simulink model "demo_ifft"  (R2023a)
settings: Solver=FixedStepDiscrete  StartTime=0.0  StopTime=dspb_ifft.SimulationTime  FixedStep=1  RelTol=1e-3  EnableMultiTasking=on
PreLoadFcn:
  | warning off Simulink:Commands:SetParamLinkChangeWarn
  | warning off Simulink:Commands:LoadMdlParameterizedLink
  | warning off Simulink:SL_SetParamLinkChangeWarn
  | warning off Simulink:SL_LoadMdlParameterizedLink
  | setup_demo_ifft;
InitFcn:
  | setup_demo_ifft;
StopFcn:
  | analyze_subchannel_fft(...
  |      dspb_ifft.FFTsize, ...
  |      dspb_ifft.subchannels, ...
  |      dspb_ifft.IFFT, ...
  |      dspb_ifft.bit_reversed, ...
  |      dspb_ifft.bit_reversed, ...
  |      v_in, chan_in,  x_in, ...
  |      v_out,chan_out, z_out);
undefined symbols (not defined in the file or in its folder): dspb_ifft, value
libraries: DSPBAPrim x8, DSPBABase x4, DSPBAVectorUtil x3, simulink x3, DspbAdvFftLibrary x2
Description:
  | This design example implements an Inverse Fast Fourier Transform.
settings Model: Creator=lrigby  LastModifiedBy=5g
settings SolverCC: AlgebraicLoopSolver=TrustRegion
settings DataIOCC: LimitDataPoints=on  SaveFormat=Array  SignalLoggingSaveFormat=ModelDataLogs  ReturnWorkspaceOutputs=off
settings OptimizationCC: ExpressionDepthLimit=2147483647  InitFltsAndDblsToZero=on  LifeSpan=inf
settings DebuggingCC: SaveWithParameterizedLinksMsg=none  UnderspecifiedInitializationDetection=Classic  MergeDetectMultiDrivingBlocksExec=none  SignalResolutionControl=TryResolveAllWithWarning  SolverPrmCheckMsg=warning  ParameterPrecisionLossMsg=none  FcnCallInpInsideContextMsg=warning  UnconnectedInputMsg=warning  UnconnectedOutputMsg=warning  UnconnectedLineMsg=warning  StateNameClashWarn=warning  SFUnexpectedBacktrackingDiag=warning  SFNoUnconditionalDefaultTransitionDiag=warning  SFExecutionAtInitializationDiag=none  ArithmeticOperatorsInVariantConditions=warning
settings HardwareCC: ProdBitPerPointer=32  ProdBitPerSizeT=32  ProdBitPerPtrDiffT=32  ProdLargestAtomicFloat=None  ProdIntDivRoundTo=Undefined  ProdEndianess=Unspecified  ProdWordSize=32  ProdHWDeviceType=ASIC/FPGA  TargetBitPerLong=64  TargetBitPerPointer=64  TargetBitPerSizeT=64  TargetBitPerPtrDiffT=64  TargetLongLongMode=on  TargetIntDivRoundTo=Zero  TargetEndianess=LittleEndian  TargetWordSize=64  TargetHWDeviceType=MATLAB Host  ProdEqTarget=off
settings ModelReferenceCC: PropagateSignalLabelsOutOfModel=off
settings SFSimCC: SimUseLocalCustomCode=off  SimParseCustomCode=off  CustomCodeUndefinedFunction=UseInterfaceOnly
settings RTWCC: RTWUseLocalCustomCode=off
settings CodeAppCC: StateflowObjectComments=on
settings GRTTargetCC: TargetFcnLib=ansi_tfl_tmw.mat  TargetLangStandard=C89/C90 (ANSI)  CombineOutputUpdateFcns=off  GRTInterface=on
settings ConfigComp: CovMetricSettings=dw  CovSaveCumulativeToWorkspaceVar=on  CovSaveSingleToWorkspaceVar=on  CovExternalEMLEnable=off

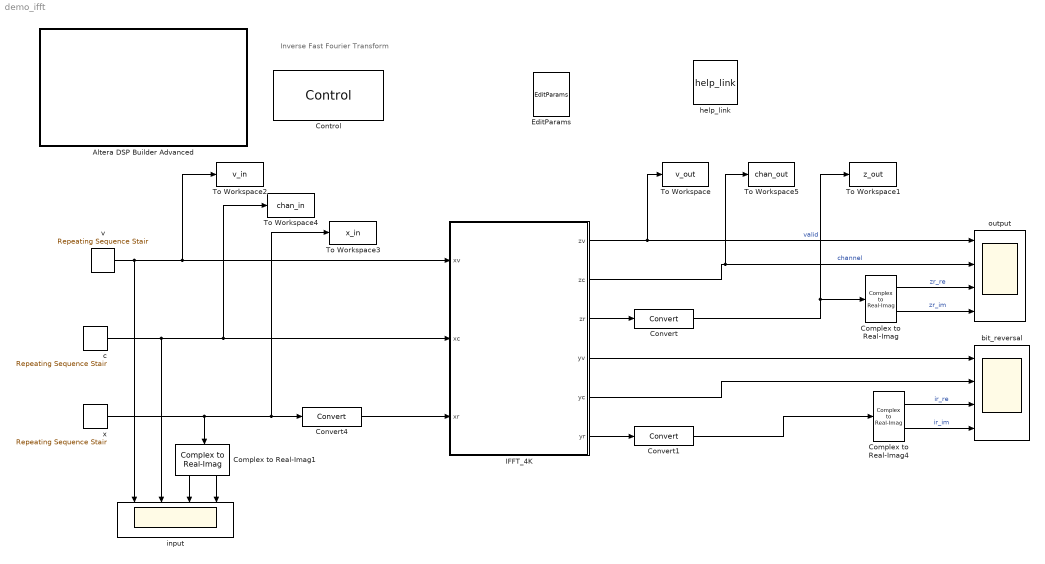
== system demo_ifft ==
  note: Inverse Fast Fourier Transform
  Altera DSP Builder Advanced : Subsystem  mask(DSP Builder Advanced Blockset Ignored Block){}
      settings: OpenFcn=web('http://www.altera.com', '-new');
      mask Display: image(imread('intellogo.tif'));
  Complex to Real-Imag : DSPBAVectorUtil/Complex to Real-Imag
  Complex to Real-Imag1 : DSPBAVectorUtil/Complex to Real-Imag
  Complex to Real-Imag4 : DSPBAVectorUtil/Complex to Real-Imag
  Control : DSPBABase/Control  generate=on  language=VHDL  destination=../rtl  make_full_path=off  path_is_relative=on  autotestbench=on  signaldepth=2  coveragetestbench=off  logs=off  spacewidth=2  spacenum=1  addrwidth=10  datawidth=16  dataendian=Big Endian  hierarchicalnames=on  ramThresholdBits=-1  distRamThresholdBits=-1  mlabThresholdBits=-1  hardMultiplierThresholdLuts=-1  version=20090407  errorOnChanMismatch=1  errorOnGPIOMismatch=0  importModelsimResults=0  cycleAccurate=off  reinterpretCastMult=off  paramFile=demo_ifft_params.xml
  Convert : DSPBAPrim/Convert  primtype=convert  nInputs=1  nOutputs=1  omode=double  otype=sfix(16)  scale=2^-15  rndmethod=Unbiased  factor=1  satmethod=None  shift_vec=[0 1 2 -1]  value=round([0:255]/17)  inPortNames=[' '; ' ';]  outPortNames=[' '; 'c']  dspbaimage=dspba_prim_wide.svg  text=fprintf('convert');  style=Optimised  visibilities=8+64+256+2^17  clipdetect=off  floatPrecision=float32_m23  advOptions=[]  version=20211007
  Convert1 : DSPBAPrim/Convert  primtype=convert  nInputs=1  nOutputs=1  omode=double  otype=sfix(16)  scale=2^-15  rndmethod=Unbiased  factor=1  satmethod=None  shift_vec=[0 1 2 -1]  value=round([0:255]/17)  inPortNames=[' '; ' ';]  outPortNames=[' '; 'c']  dspbaimage=dspba_prim_wide.svg  text=fprintf('convert');  style=Optimised  visibilities=8+64+256+2^17  clipdetect=off  floatPrecision=float32_m23  advOptions=[]  version=20211007
  Convert4 : DSPBAPrim/Convert  primtype=convert  nInputs=1  nOutputs=1  omode=Specify via dialog  otype=sfix(16)  scale=2^-14  rndmethod=Unbiased  factor=1  satmethod=None  shift_vec=[0 1 2 -1]  value=round([0:255]/17)  inPortNames=[' '; ' ';]  outPortNames=[' '; 'c']  dspbaimage=dspba_prim_wide.svg  text=fprintf('convert');  style=Optimised  visibilities=8+64+256+2^17  clipdetect=off  floatPrecision=float32_m23  advOptions=[]  version=20211007
  EditParams : DSPBABase/EditParams  version=20090407
  IFFT_4K : Subsystem
  To Workspace : ToWorkspace  VariableName=v_out  SampleTime=-1
  To Workspace1 : ToWorkspace  VariableName=z_out  SampleTime=-1
  To Workspace2 : ToWorkspace  VariableName=v_in  SampleTime=-1
  To Workspace3 : ToWorkspace  VariableName=x_in  SampleTime=-1
  To Workspace4 : ToWorkspace  VariableName=chan_in  SampleTime=-1
  To Workspace5 : ToWorkspace  VariableName=chan_out  SampleTime=-1
  bit_reversal : Scope  NumInputPorts=4
  c : simulink/Sources/Repeating Sequence Stair  OutValues=dspb_ifft.channel_in  tsamp=dspb_ifft.SampleTime  OutMin=[]  OutMax=[]  OutDataTypeStr=fixdt(0,8,0)  OutputDataTypeScalingMode=Specify via dialog  OutDataType=uint(8)  ConRadixGroup=Use specified scaling  OutScaling=2^-15
  help_link : DSPBABase/help_link  version=20090407
  input : Scope  NumInputPorts=4
  output : Scope  NumInputPorts=4
  v : simulink/Sources/Repeating Sequence Stair  OutValues=dspb_ifft.valid_in  tsamp=dspb_ifft.SampleTime  OutMin=[]  OutMax=[]  OutDataTypeStr=fixdt('boolean')  OutputDataTypeScalingMode=Specify via dialog  OutDataType=fixdt('boolean')  ConRadixGroup=Best Precision: Vector-wise  OutScaling=[]
  x : simulink/Sources/Repeating Sequence Stair  OutValues=dspb_ifft.x_in  tsamp=dspb_ifft.SampleTime  OutMin=[]  OutMax=[]  OutDataTypeStr=double  OutputDataTypeScalingMode=double  OutDataType=dspb_ifft.InputType  ConRadixGroup=Best Precision: Vector-wise  OutScaling=[]
  wires:
  v/1 -> input/1, To Workspace2/1, IFFT_4K/1(xv)
  c/1 -> To Workspace4/1, IFFT_4K/2(xc), input/2
  x/1 -> Complex to Real-Imag1/1, To Workspace3/1, Convert4/1
  IFFT_4K/3(zr) -> Convert/1
  Complex to Real-Imag/1 -> output/3  "zr_re"
  Complex to Real-Imag/2 -> output/4  "zr_im"
  Complex to Real-Imag1/1 -> input/3
  Complex to Real-Imag1/2 -> input/4
  Convert/1 -> Complex to Real-Imag/1, To Workspace1/1
  IFFT_4K/6(yr) -> Convert1/1
  IFFT_4K/1(zv) -> output/1, To Workspace/1  "valid"
  IFFT_4K/2(zc) -> output/2, To Workspace5/1  "channel"
  Convert4/1 -> IFFT_4K/3(xr)
  Convert1/1 -> Complex to Real-Imag4/1
  IFFT_4K/4(yv) -> bit_reversal/1
  IFFT_4K/5(yc) -> bit_reversal/2
  Complex to Real-Imag4/1 -> bit_reversal/3  "ir_re"
  Complex to Real-Imag4/2 -> bit_reversal/4  "ir_im"

== system demo_ifft/Altera DSP Builder Advanced ==

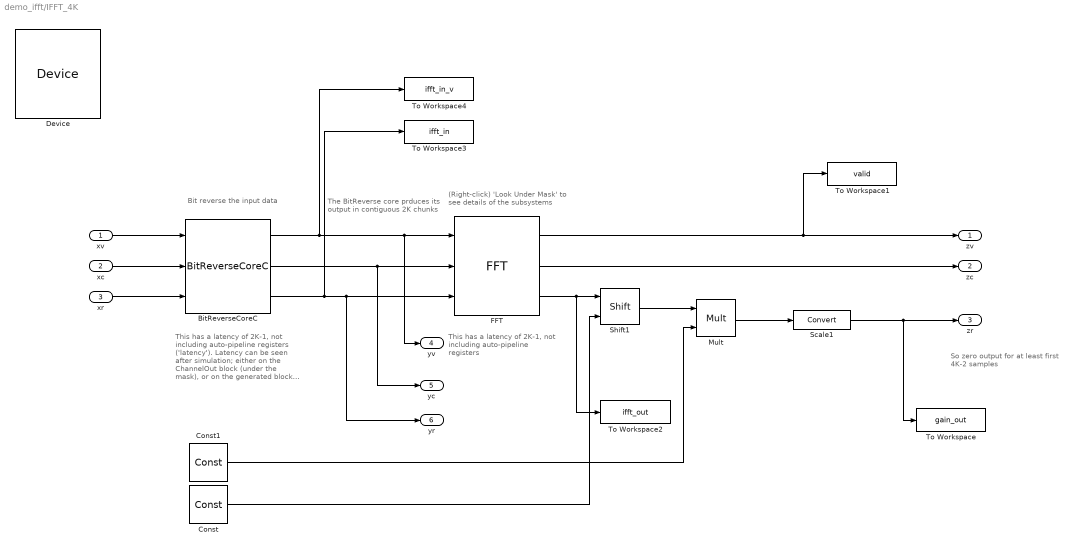
== system demo_ifft/IFFT_4K ==
  note: Bit reverse the input data
  note: This has a latency of 2K-1,
      | not including auto-pipeline
      | registers ('latency'). Latency
      | can be seen after simulation;
      | either on the ChannelOut block
      | (under the mask), or on the
      | generated block help.
  note: This has a latency of 2K-1,
      | not including auto-pipeline
      | registers
  note: So zero output for at
      | least first 4K-2 samples
  note: (Right-click) 'Look Under Mask'
      | to see details of the subsystems
  note: The BitReverse core prduces its
      | output in contiguous 2K chunks
  xv : Inport
  xc : Inport  Port=2
  xr : Inport  Port=3
  BitReverseCoreC : DspbAdvFftLibrary/Radix2/BitReverseCoreC  N=dspb_ifft.FFTsize  subchannels=dspb_ifft.subchannels
      link override ChannelOut: value=1  latency=6  nInputs=dspba_internal_get_channel_ports(gcb, 'inputs')  nOutputs=dspba_internal_get_channel_ports(gcb, 'outputs')  packetBeginEnabled=off  version=20140818
  Const : DSPBAPrim/Const  primtype=const  nInputs=0  nOutputs=1  omode=Specify via dialog  otype=ufix(4)  scale=0  rndmethod=Unbiased  factor=1  satmethod=Symmetric  shift_vec=[0 1 2 -1]  value=12  inPortNames=['+'; '+';]  outPortNames=[' ']  dspbaimage=dspba_prim.svg  text=fprintf('%s', num2str(value));  style=Optimised  visibilities=8 + 1024  floatPrecision=float32_m23  warnSaturation=on  version=20211007  SampleTime=inf
  Const1 : DSPBAPrim/Const  primtype=const  nInputs=0  nOutputs=1  omode=Specify via dialog  otype=sfix(16)  scale=2^-13  rndmethod=Unbiased  factor=1  satmethod=Symmetric  shift_vec=[0 1 2 -1]  value=1  inPortNames=['+'; '+';]  outPortNames=[' ']  dspbaimage=dspba_prim.svg  text=fprintf('%s', num2str(value));  style=Optimised  visibilities=8 + 1024  floatPrecision=float32_m23  warnSaturation=on  version=20211007  SampleTime=inf
  Device : DSPBABase/Device  family=Arria 10  stratix4device=Stratix IV E  hardcopy4device=HardCopy IV E  stratix5device=Stratix V GX  device=AUTO  speed=-3  stratixSpeed=-5  stratix2Speed=-3  stratix3Speed=-3  stratix4gxSpeed=-2  stratix4gtSpeed=-1  cyclone2Speed=-6  cyclone3Speed=-6  arria2Speed=-4  cyclone4eSpeed=-8  stratix5Speed=-3  arria5Speed=-4  arriaSpeed=-6  cyclone3lsSpeed=-7  cyclone5Speed=-6  arria2gzSpeed=-3  nightFurySpeed=-2  ecp2Speed=-7  hardcopycompat=off  version=20140217  max10flashmode=off  max10nomeminit=off
  FFT : DspbAdvFftLibrary/Common/FFT  IFFT=dspb_ifft.IFFT  subchannels=dspb_ifft.subchannels  br_in=~dspb_ifft.bit_reversed  N=dspb_ifft.N  in_type=dspb_ifft.input_type  type_strings=dspb_ifft.type_strings  faithful=true
      link override ChannelOut1: nInputs=dspba_internal_get_channel_ports(gcb, 'inputs')  nOutputs=dspba_internal_get_channel_ports(gcb, 'outputs')  value=1  packetBeginEnabled=off  latency=34  version=20140818
  Mult : DSPBAPrim/Mult  primtype=mult  nInputs=2  nOutputs=1  omode=Inherit via internal rule  otype=sfix(16)  scale=2^-15  rndmethod=Unbiased  factor=1  satmethod=Symmetric  shift_vec=[0 1 2 -1]  value=0  inPortNames=[' '; ' ';]  outPortNames=[' ']  dspbaimage=dspba_prim.svg  text=fprintf('X');  style=Optimised  visibilities=8+2^18+2^19  floatPrecision=float32_m23  floatRounding=correct  advOptions=[]  version=20211007
  Scale1 : DSPBAPrim/Convert  primtype=convert  nInputs=1  nOutputs=1  omode=Specify via dialog  otype=sfix(16)  scale=2^-14  rndmethod=Biased  factor=1  satmethod=Symmetric  shift_vec=[0 1 2 -1]  value=round([0:255]/17)  inPortNames=[' '; ' ';]  outPortNames=[' '; 'c']  dspbaimage=dspba_prim_wide.svg  text=fprintf('convert');  style=Optimised  visibilities=8+64+256+2^17  clipdetect=off  floatPrecision=float32_m23  advOptions=[]  version=20211007
  Shift1 : DSPBAPrim/Shift  primtype=shift  nInputs=2  nOutputs=1  omode=Inherit via internal rule  otype=sfix(16)  scale=2^-15  rndmethod=Unbiased  factor=1  satmethod=Symmetric  shift_vec=[0 1 2 -1]  value=0  inPortNames=['a'; 'b';]  outPortNames=[' ']  dspbaimage=dspba_prim.svg  text=fprintf('a >> b');  style=Optimised  visibilities=8  version=20211007
  To Workspace : ToWorkspace  VariableName=gain_out  SampleTime=-1
      settings: Save2DSignal=2-D array (concatenate along first dimension)
  To Workspace1 : ToWorkspace  VariableName=valid  SampleTime=-1
      settings: Save2DSignal=2-D array (concatenate along first dimension)
  To Workspace2 : ToWorkspace  VariableName=ifft_out  SampleTime=-1
      settings: Save2DSignal=2-D array (concatenate along first dimension)
  To Workspace3 : ToWorkspace  VariableName=ifft_in  SampleTime=-1
      settings: Save2DSignal=2-D array (concatenate along first dimension)
  To Workspace4 : ToWorkspace  VariableName=ifft_in_v  SampleTime=-1
      settings: Save2DSignal=2-D array (concatenate along first dimension)
  zv : Outport
  zc : Outport  Port=2
  zr : Outport  Port=3
  yv : Outport  Port=4
  yc : Outport  Port=5
  yr : Outport  Port=6
  wires:
  BitReverseCoreC/1 -> To Workspace4/1, FFT/1, yv/1
  BitReverseCoreC/2 -> FFT/2, yc/1
  BitReverseCoreC/3 -> FFT/3, yr/1, To Workspace3/1
  FFT/2 -> zc/1
  FFT/1 -> To Workspace1/1, zv/1
  FFT/3 -> Shift1/1, To Workspace2/1
  Mult/1 -> Scale1/1
  Shift1/1 -> Mult/1
  Const1/1 -> Mult/2
  Const/1 -> Shift1/2
  Scale1/1 -> zr/1, To Workspace/1
  xv/1 -> BitReverseCoreC/1
  xc/1 -> BitReverseCoreC/2
  xr/1 -> BitReverseCoreC/3
